simulink model "CRH2forBenchmark"  (R2014a)
settings: Solver=ode3  StartTime=0.0  StopTime=1  FixedStep=1e-5  RelTol=1e-3
PostLoadFcn:
  | , if any(exist('dsrtsu_mdlpostloadfcn', 'file') == [2, 3, 6]), try dsrtsu_mdlpostloadfcn('Execute', bdroot); catch fprintf('Error in PostLoadFcn (dsrtsu_mdlpostloadfcn) for model "%s":\n %s\n', bdroot, lasterr); end, end,
values from neighbouring files (symbols this model uses):
  Cd = 0.016    [CRH2forBenchmark.mat]
  Lm = 0.032848    [CRH2forBenchmark.mat]
  Ln = 0.002    [CRH2forBenchmark.mat]
  Lr = 0.034142    [CRH2forBenchmark.mat]
  Ls = 0.0342654    [CRH2forBenchmark.mat]
  np = 2    [CRH2forBenchmark.mat]
  Rd = 6000    [CRH2forBenchmark.mat]
  Rn = 0.2    [CRH2forBenchmark.mat]
  Rr = 0.146    [CRH2forBenchmark.mat]
  Rs = 0.144    [CRH2forBenchmark.mat]
  ts = 1e-05    [CRH2forBenchmark.mat]
undefined symbols (not defined in the file): J, KIM, KIT, KPM, KPT, phir, Ts, Vge
libraries: simulink x10
(part 2 of 3)

== system CRH2forBenchmark/InverterN/InverterTuN ==
  Tu1 : Inport
  Tu2 : Inport  Port=2
  Tu3 : Inport  Port=3
  Tu4 : Inport  Port=4
  Ia : Inport  Port=5
  U1 : Inport  Port=6
  U2 : Inport  Port=7
  InverterTuN_sfcn : S-Function  FunctionName=InverterTuN_sf  SFunctionModules=""  EnableBusSupport=off  mask{rtw_sf_name=InverterTuN_sf, showVar=off}
      mask prompts: rtw_sf_name "Simulink:masks:GenSFuncName_MP"; showVar "Simulink:masks:GenSFuncShowModuleList_MP"
      mask help: Simulink:masks:GenSFuncDesc_MD
      mask init: same as CRH2forBenchmark/DCU1/DCU1_sfcn
      settings: CopyFcn=|
      | if ~strcmp(get_param(gcb,'Linkstatus'),'none') && ...
      | ~strcmp(get_param(gcb,'Linkstatus'),'implicit')
      |   set_param(gcb,'LinkStatus','none');
      | end
      mask Help: eval('feval(''rtwprivate'',''rtwhelpview'',''rtw_sfcn_block'')');
      mask Display:
      | port_label('input',1,'Tu1');
      | port_label('input',2,'Tu2');
      | port_label('input',3,'Tu3');
      | port_label('input',4,'Tu4');
      | port_label('input',5,'Ia');
      | port_label('input',6,'U1');
      | port_label('input',7,'U2');
      | port_label('output',1,'Iu');
      | port_label('output',2,'Iz');
      | port_label('output',3,'Id');
      | port_label('output',4,'Vu');
  __InputSSForSFun__ : Subsystem
  __OutputSSForSFun__ : Subsystem
  Iu : Outport
  Iz : Outport  Port=2
  Id : Outport  Port=3
  Vu : Outport  Port=4
  wires:
  Tu1/1 -> __InputSSForSFun__/1(Tu1)
  Tu2/1 -> __InputSSForSFun__/2(Tu2)
  Tu3/1 -> __InputSSForSFun__/3(Tu3)
  Tu4/1 -> __InputSSForSFun__/4(Tu4)
  Ia/1 -> __InputSSForSFun__/5(Ia)
  U1/1 -> __InputSSForSFun__/6(U1)
  U2/1 -> __InputSSForSFun__/7(U2)
  __InputSSForSFun__/1(__UniqueOutportName__1__) -> InverterTuN_sfcn/1
  __InputSSForSFun__/2(__UniqueOutportName__2__) -> InverterTuN_sfcn/2
  __InputSSForSFun__/3(__UniqueOutportName__3__) -> InverterTuN_sfcn/3
  __InputSSForSFun__/4(__UniqueOutportName__4__) -> InverterTuN_sfcn/4
  __InputSSForSFun__/5(__UniqueOutportName__5__) -> InverterTuN_sfcn/5
  __InputSSForSFun__/6(__UniqueOutportName__6__) -> InverterTuN_sfcn/6
  __InputSSForSFun__/7(__UniqueOutportName__7__) -> InverterTuN_sfcn/7
  InverterTuN_sfcn/1 -> __OutputSSForSFun__/1(__UniqueInportName__1__)
  InverterTuN_sfcn/2 -> __OutputSSForSFun__/2(__UniqueInportName__2__)
  InverterTuN_sfcn/3 -> __OutputSSForSFun__/3(__UniqueInportName__3__)
  InverterTuN_sfcn/4 -> __OutputSSForSFun__/4(__UniqueInportName__4__)
  __OutputSSForSFun__/1(Iu) -> Iu/1
  __OutputSSForSFun__/2(Iz) -> Iz/1
  __OutputSSForSFun__/3(Id) -> Id/1
  __OutputSSForSFun__/4(Vu) -> Vu/1

== system CRH2forBenchmark/InverterN/InverterTvN ==
  Tv1 : Inport
  Tv2 : Inport  Port=2
  Tv3 : Inport  Port=3
  Tv4 : Inport  Port=4
  Ib : Inport  Port=5
  U1 : Inport  Port=6
  U2 : Inport  Port=7
  InverterTvN_sfcn : S-Function  FunctionName=InverterTvN_sf  SFunctionModules=""  EnableBusSupport=off  mask{rtw_sf_name=InverterTvN_sf, showVar=off}
      mask prompts: rtw_sf_name "Simulink:masks:GenSFuncName_MP"; showVar "Simulink:masks:GenSFuncShowModuleList_MP"
      mask help: Simulink:masks:GenSFuncDesc_MD
      mask init: same as CRH2forBenchmark/DCU1/DCU1_sfcn
      settings: CopyFcn=|
      | if ~strcmp(get_param(gcb,'Linkstatus'),'none') && ...
      | ~strcmp(get_param(gcb,'Linkstatus'),'implicit')
      |   set_param(gcb,'LinkStatus','none');
      | end
      mask Help: eval('feval(''rtwprivate'',''rtwhelpview'',''rtw_sfcn_block'')');
      mask Display:
      | port_label('input',1,'Tv1');
      | port_label('input',2,'Tv2');
      | port_label('input',3,'Tv3');
      | port_label('input',4,'Tv4');
      | port_label('input',5,'Ib');
      | port_label('input',6,'U1');
      | port_label('input',7,'U2');
      | port_label('output',1,'Iu');
      | port_label('output',2,'Iz');
      | port_label('output',3,'Id');
      | port_label('output',4,'Vv');
  __InputSSForSFun__ : Subsystem
  __OutputSSForSFun__ : Subsystem
  Iu : Outport
  Iz : Outport  Port=2
  Id : Outport  Port=3
  Vv : Outport  Port=4
  wires:
  Tv1/1 -> __InputSSForSFun__/1(Tv1)
  Tv2/1 -> __InputSSForSFun__/2(Tv2)
  Tv3/1 -> __InputSSForSFun__/3(Tv3)
  Tv4/1 -> __InputSSForSFun__/4(Tv4)
  Ib/1 -> __InputSSForSFun__/5(Ib)
  U1/1 -> __InputSSForSFun__/6(U1)
  U2/1 -> __InputSSForSFun__/7(U2)
  __InputSSForSFun__/1(__UniqueOutportName__1__) -> InverterTvN_sfcn/1
  __InputSSForSFun__/2(__UniqueOutportName__2__) -> InverterTvN_sfcn/2
  __InputSSForSFun__/3(__UniqueOutportName__3__) -> InverterTvN_sfcn/3
  __InputSSForSFun__/4(__UniqueOutportName__4__) -> InverterTvN_sfcn/4
  __InputSSForSFun__/5(__UniqueOutportName__5__) -> InverterTvN_sfcn/5
  __InputSSForSFun__/6(__UniqueOutportName__6__) -> InverterTvN_sfcn/6
  __InputSSForSFun__/7(__UniqueOutportName__7__) -> InverterTvN_sfcn/7
  InverterTvN_sfcn/1 -> __OutputSSForSFun__/1(__UniqueInportName__1__)
  InverterTvN_sfcn/2 -> __OutputSSForSFun__/2(__UniqueInportName__2__)
  InverterTvN_sfcn/3 -> __OutputSSForSFun__/3(__UniqueInportName__3__)
  InverterTvN_sfcn/4 -> __OutputSSForSFun__/4(__UniqueInportName__4__)
  __OutputSSForSFun__/1(Iu) -> Iu/1
  __OutputSSForSFun__/2(Iz) -> Iz/1
  __OutputSSForSFun__/3(Id) -> Id/1
  __OutputSSForSFun__/4(Vv) -> Vv/1

== system CRH2forBenchmark/InverterN/InverterTwN ==
  Tw1 : Inport
  Tw2 : Inport  Port=2
  Tw3 : Inport  Port=3
  Tw4 : Inport  Port=4
  Ic : Inport  Port=5
  U1 : Inport  Port=6
  U2 : Inport  Port=7
  InverterTwN_sfcn : S-Function  FunctionName=InverterTwN_sf  SFunctionModules=""  EnableBusSupport=off  mask{rtw_sf_name=InverterTwN_sf, showVar=off}
      mask prompts: rtw_sf_name "Simulink:masks:GenSFuncName_MP"; showVar "Simulink:masks:GenSFuncShowModuleList_MP"
      mask help: Simulink:masks:GenSFuncDesc_MD
      mask init: same as CRH2forBenchmark/DCU1/DCU1_sfcn
      settings: CopyFcn=|
      | if ~strcmp(get_param(gcb,'Linkstatus'),'none') && ...
      | ~strcmp(get_param(gcb,'Linkstatus'),'implicit')
      |   set_param(gcb,'LinkStatus','none');
      | end
      mask Help: eval('feval(''rtwprivate'',''rtwhelpview'',''rtw_sfcn_block'')');
      mask Display:
      | port_label('input',1,'Tw1');
      | port_label('input',2,'Tw2');
      | port_label('input',3,'Tw3');
      | port_label('input',4,'Tw4');
      | port_label('input',5,'Ic');
      | port_label('input',6,'U1');
      | port_label('input',7,'U2');
      | port_label('output',1,'Iu');
      | port_label('output',2,'Iz');
      | port_label('output',3,'Id');
      | port_label('output',4,'Vw');
  __InputSSForSFun__ : Subsystem
  __OutputSSForSFun__ : Subsystem
  Iu : Outport
  Iz : Outport  Port=2
  Id : Outport  Port=3
  Vw : Outport  Port=4
  wires:
  Tw1/1 -> __InputSSForSFun__/1(Tw1)
  Tw2/1 -> __InputSSForSFun__/2(Tw2)
  Tw3/1 -> __InputSSForSFun__/3(Tw3)
  Tw4/1 -> __InputSSForSFun__/4(Tw4)
  Ic/1 -> __InputSSForSFun__/5(Ic)
  U1/1 -> __InputSSForSFun__/6(U1)
  U2/1 -> __InputSSForSFun__/7(U2)
  __InputSSForSFun__/1(__UniqueOutportName__1__) -> InverterTwN_sfcn/1
  __InputSSForSFun__/2(__UniqueOutportName__2__) -> InverterTwN_sfcn/2
  __InputSSForSFun__/3(__UniqueOutportName__3__) -> InverterTwN_sfcn/3
  __InputSSForSFun__/4(__UniqueOutportName__4__) -> InverterTwN_sfcn/4
  __InputSSForSFun__/5(__UniqueOutportName__5__) -> InverterTwN_sfcn/5
  __InputSSForSFun__/6(__UniqueOutportName__6__) -> InverterTwN_sfcn/6
  __InputSSForSFun__/7(__UniqueOutportName__7__) -> InverterTwN_sfcn/7
  InverterTwN_sfcn/1 -> __OutputSSForSFun__/1(__UniqueInportName__1__)
  InverterTwN_sfcn/2 -> __OutputSSForSFun__/2(__UniqueInportName__2__)
  InverterTwN_sfcn/3 -> __OutputSSForSFun__/3(__UniqueInportName__3__)
  InverterTwN_sfcn/4 -> __OutputSSForSFun__/4(__UniqueInportName__4__)
  __OutputSSForSFun__/1(Iu) -> Iu/1
  __OutputSSForSFun__/2(Iz) -> Iz/1
  __OutputSSForSFun__/3(Id) -> Id/1
  __OutputSSForSFun__/4(Vw) -> Vw/1

== system CRH2forBenchmark/InverterN/Pulse ==
  note: PhaseA:1 to 4
      |
      | PhaseB:5 to 8
      |
      | PhaseC:9 to 12
  State : Inport
  Add : Sum
  Constant : Constant  Value=2
  Demux : Demux  Outputs=3
  Multiport Switch : MultiPortSwitch
  Multiport Switch1 : MultiPortSwitch
  Multiport Switch2 : MultiPortSwitch
  Mux : Mux  Inputs=3
  S =  Ud : Constant  Value=[1 1 0 0]
  S = - Ud : Constant  Value=[0 0 1 1]
  S = 0 : Constant  Value=[0 1 1 0]
  SVPWM : Outport
  wires:
  S = - Ud/1 -> Multiport Switch2/2, Multiport Switch/2, Multiport Switch1/2
  Multiport Switch/1 -> Mux/1
  S =  Ud/1 -> Multiport Switch2/4, Multiport Switch1/4, Multiport Switch/4
  Multiport Switch2/1 -> Mux/3
  Demux/1 -> Multiport Switch/1
  Mux/1 -> SVPWM/1
  Constant/1 -> Add/2
  State/1 -> Add/1
  Demux/3 -> Multiport Switch2/1
  Demux/2 -> Multiport Switch1/1
  S = 0/1 -> Multiport Switch2/3, Multiport Switch1/3, Multiport Switch/3
  Multiport Switch1/1 -> Mux/2
  Add/1 -> Demux/1

== system CRH2forBenchmark/Machine model/Normal ModelF ==
  Ua : Inport
  Ub : Inport  Port=2
  Uc : Inport  Port=3
  TL : Inport  Port=4
  MeasurementF : Subsystem  mask{sfcnParam1=J, sfcnParam2=Lm, sfcnParam3=np}
      mask prompts: sfcnParam1 "J:"; sfcnParam2 "Lm:"; sfcnParam3 "np:"
      mask help: Simulink:masks:GenSFuncDesc_MD
      mask Help: eval('feval(''rtwprivate'',''rtwhelpview'',''rtw_sfcn_block'')');
  MotorSubsystem1F : Subsystem
  MotorSubsystem2F : Subsystem
  MotorSubsystem3F : Subsystem
  MotorSubsystemF : Subsystem
  r2sF : Subsystem
      mask help: Simulink:masks:GenSFuncDesc_MD
      mask Help: eval('feval(''rtwprivate'',''rtwhelpview'',''rtw_sfcn_block'')');
  Te0 : Outport
  Isabc0 : Outport  Port=2
  w : Outport  Port=3
  wires:
  MeasurementF/3(Isabc) -> Isabc0/1
  MotorSubsystem2F/2(ψrα) -> MotorSubsystem3F/2(ψrα), MotorSubsystemF/1(ψrα)
  MotorSubsystem1F/2(ψsβ) -> MotorSubsystem3F/1(ψsβ)
  MotorSubsystem2F/1(irα) -> MeasurementF/3(irα)
  MeasurementF/1(Te) -> Te0/1
  TL/1 -> MeasurementF/5(TL)
  MotorSubsystemF/2(ψsα) -> MotorSubsystem2F/1(ψsα)
  r2sF/1(Usα) -> MotorSubsystemF/2(Usα)
  MotorSubsystem3F/2(ψrβ) -> MotorSubsystem1F/1(ψrβ), MotorSubsystem2F/2(ψrβ)
  MotorSubsystemF/1(isα) -> MeasurementF/1(isα)
  r2sF/2(Usβ) -> MotorSubsystem1F/2(Usβ)
  MotorSubsystem3F/1(irβ) -> MeasurementF/4(irβ)
  MeasurementF/2(ω) -> MotorSubsystem2F/3(ω), MotorSubsystem3F/3(ω), w/1
  MotorSubsystem1F/1(isβ) -> MeasurementF/2(isβ)
  Uc/1 -> r2sF/3(Uc)
  Ub/1 -> r2sF/2(Ub)
  Ua/1 -> r2sF/1(Ua)

== system CRH2forBenchmark/Machine model1/Normal ModelN ==
  Ua : Inport
  Ub : Inport  Port=2
  Uc : Inport  Port=3
  TL : Inport  Port=4
  MeasurementN : Subsystem  mask{sfcnParam1=J, sfcnParam2=Lm, sfcnParam3=np}
      mask prompts: sfcnParam1 "J:"; sfcnParam2 "Lm:"; sfcnParam3 "np:"
      mask help: Simulink:masks:GenSFuncDesc_MD
      mask Help: eval('feval(''rtwprivate'',''rtwhelpview'',''rtw_sfcn_block'')');
  MotorSubsystem1N : Subsystem
  MotorSubsystem2N : Subsystem
  MotorSubsystem3N : Subsystem
  MotorSubsystemN : Subsystem
  r2sN : Subsystem
      mask help: Simulink:masks:GenSFuncDesc_MD
      mask Help: eval('feval(''rtwprivate'',''rtwhelpview'',''rtw_sfcn_block'')');
  Te0 : Outport
  Isabc0 : Outport  Port=2
  w : Outport  Port=3
  wires:
  MeasurementN/3(Isabc) -> Isabc0/1
  MotorSubsystem2N/2(ψrα) -> MotorSubsystem3N/2(ψrα), MotorSubsystemN/1(ψrα)
  MotorSubsystem1N/2(ψsβ) -> MotorSubsystem3N/1(ψsβ)
  MotorSubsystem2N/1(irα) -> MeasurementN/3(irα)
  MeasurementN/1(Te) -> Te0/1
  TL/1 -> MeasurementN/5(TL)
  MotorSubsystemN/2(ψsα) -> MotorSubsystem2N/1(ψsα)
  r2sN/1(Usα) -> MotorSubsystemN/2(Usα)
  MotorSubsystem3N/2(ψrβ) -> MotorSubsystem1N/1(ψrβ), MotorSubsystem2N/2(ψrβ)
  MotorSubsystemN/1(isα) -> MeasurementN/1(isα)
  r2sN/2(Usβ) -> MotorSubsystem1N/2(Usβ)
  MotorSubsystem3N/1(irβ) -> MeasurementN/4(irβ)
  MeasurementN/2(ω) -> MotorSubsystem2N/3(ω), MotorSubsystem3N/3(ω), w/1
  MotorSubsystem1N/1(isβ) -> MeasurementN/2(isβ)
  Uc/1 -> r2sN/3(Uc)
  Ub/1 -> r2sN/2(Ub)
  Ua/1 -> r2sN/1(Ua)

== system CRH2forBenchmark/TFI1/TFI1Sub ==
  Nomal : Inport
  Outside Signal : Inport  Port=2
  Add : Sum
  Band-Limited White Noise : simulink/Sources/Band-Limited White Noise  Cov=NoiseFault(1)  Ts=NoiseFault(2)  seed=NoiseFault(3)
  Logic Operation : Subsystem
  Noise0 : Constant  Value=0
  NoiseAdd : Sum  Inputs=++|
  NoiseSelec : Constant  Value=NoiseSelec
  Product : Product
  Switch : Switch  Criteria=u2 ~= 0
  TFI : Subsystem
  Out : Outport
  wires:
  NoiseSelec/1 -> Switch/2
  [Selector] -> Logic Operation/1(Selector)
  TFI/2(Selector) -> [Selector]
  Product/1 -> Logic Operation/3(Mux)
  TFI/1(Fault Singal) -> [Fault]
  Noise0/1 -> Switch/3
  Add/1 -> Logic Operation/2(Add)
  Nomal/1 -> Logic Operation/4(Normal), Product/1, Add/1
  Logic Operation/1(Out) -> NoiseAdd/2
  NoiseAdd/1 -> Out/1
  [Fault] -> Product/2, Add/2, Logic Operation/5(Fault)
  Band-Limited White Noise/1 -> Switch/1
  Switch/1 -> NoiseAdd/1
  Outside Signal/1 -> TFI/1(Outside Signal)

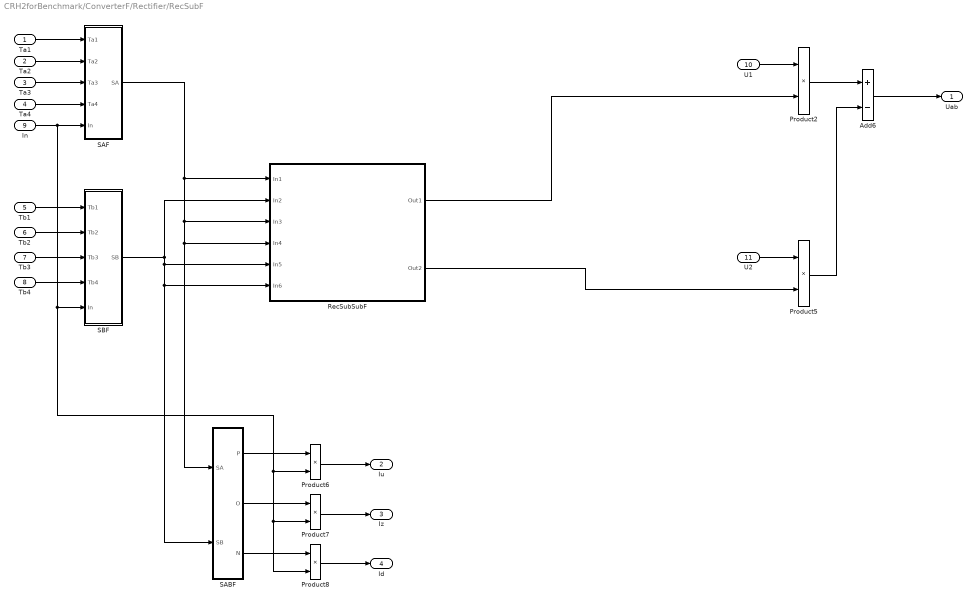
== system CRH2forBenchmark/ConverterF/Rectifier/RecSubF ==
  Ta1 : Inport
  Ta2 : Inport  Port=2
  Ta3 : Inport  Port=3
  Ta4 : Inport  Port=4
  Tb1 : Inport  Port=5
  Tb2 : Inport  Port=6
  Tb3 : Inport  Port=7
  Tb4 : Inport  Port=8
  In : Inport  Port=9
  U1 : Inport  Port=10
  U2 : Inport  Port=11
  Add6 : Sum  Inputs=+-  SampleTime=ts
  Product{2,5..8} (5 alike) : Product  SampleTime=ts
  RecSubSubF : Subsystem
      mask help: Simulink:masks:GenSFuncDesc_MD
      mask Help: eval('feval(''rtwprivate'',''rtwhelpview'',''rtw_sfcn_block'')');
  SABF : Subsystem
      mask help: Simulink:masks:GenSFuncDesc_MD
      mask Help: eval('feval(''rtwprivate'',''rtwhelpview'',''rtw_sfcn_block'')');
  SAF : Subsystem
      mask help: Simulink:masks:GenSFuncDesc_MD
      mask Help: eval('feval(''rtwprivate'',''rtwhelpview'',''rtw_sfcn_block'')');
  SBF : Subsystem
      mask help: Simulink:masks:GenSFuncDesc_MD
      mask Help: eval('feval(''rtwprivate'',''rtwhelpview'',''rtw_sfcn_block'')');
  Uab : Outport
  Iu : Outport  Port=2
  Iz : Outport  Port=3
  Id : Outport  Port=4
  wires:
  In/1 -> SAF/5(In), SBF/5(In), Product7/2, Product8/2, Product6/2
  Tb3/1 -> SBF/3(Tb3)
  U2/1 -> Product5/1
  Product2/1 -> Add6/1
  SAF/1(SA) -> RecSubSubF/1(In1), RecSubSubF/3(In3), RecSubSubF/4(In4), SABF/1(SA)
  U1/1 -> Product2/1
  Ta3/1 -> SAF/3(Ta3)
  Product5/1 -> Add6/2
  Tb1/1 -> SBF/1(Tb1)
  Add6/1 -> Uab/1
  Ta2/1 -> SAF/2(Ta2)
  Tb2/1 -> SBF/2(Tb2)
  SBF/1(SB) -> RecSubSubF/2(In2), RecSubSubF/5(In5), RecSubSubF/6(In6), SABF/2(SB)
  Tb4/1 -> SBF/4(Tb4)
  Ta1/1 -> SAF/1(Ta1)
  Ta4/1 -> SAF/4(Ta4)
  SABF/3(N) -> Product8/1
  SABF/2(O) -> Product7/1
  SABF/1(P) -> Product6/1
  Product6/1 -> Iu/1
  Product7/1 -> Iz/1
  Product8/1 -> Id/1
  RecSubSubF/1(Out1) -> Product2/2
  RecSubSubF/2(Out2) -> Product5/2

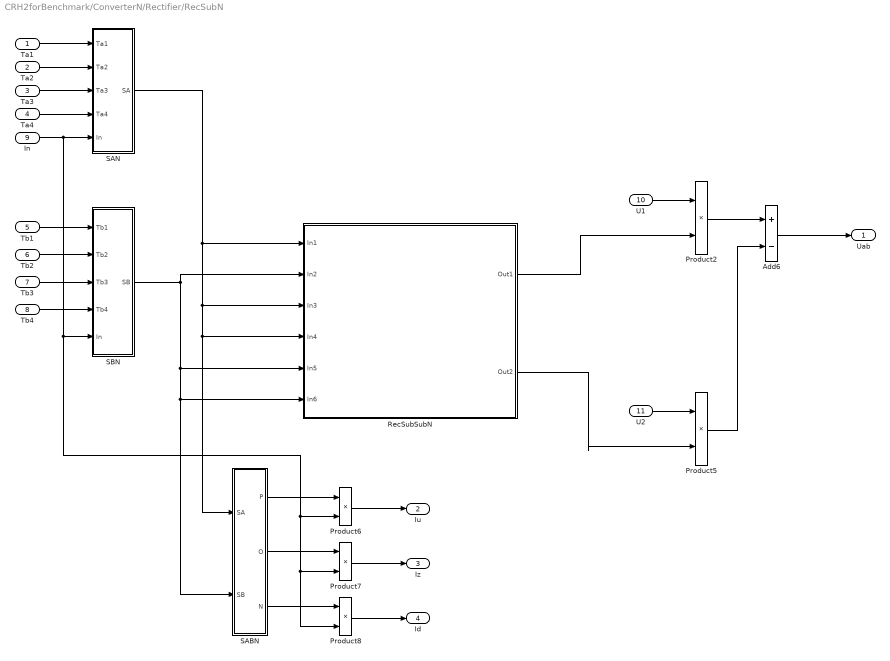
== system CRH2forBenchmark/ConverterN/Rectifier/RecSubN ==
  Ta1 : Inport
  Ta2 : Inport  Port=2
  Ta3 : Inport  Port=3
  Ta4 : Inport  Port=4
  Tb1 : Inport  Port=5
  Tb2 : Inport  Port=6
  Tb3 : Inport  Port=7
  Tb4 : Inport  Port=8
  In : Inport  Port=9
  U1 : Inport  Port=10
  U2 : Inport  Port=11
  Add6 : Sum  Inputs=+-  SampleTime=ts
  Product{2,5..8} (5 alike) : Product  SampleTime=ts
  RecSubSubN : Subsystem
      mask help: Simulink:masks:GenSFuncDesc_MD
      mask Help: eval('feval(''rtwprivate'',''rtwhelpview'',''rtw_sfcn_block'')');
  SABN : Subsystem
      mask help: Simulink:masks:GenSFuncDesc_MD
      mask Help: eval('feval(''rtwprivate'',''rtwhelpview'',''rtw_sfcn_block'')');
  SAN : Subsystem
      mask help: Simulink:masks:GenSFuncDesc_MD
      mask Help: eval('feval(''rtwprivate'',''rtwhelpview'',''rtw_sfcn_block'')');
  SBN : Subsystem
      mask help: Simulink:masks:GenSFuncDesc_MD
      mask Help: eval('feval(''rtwprivate'',''rtwhelpview'',''rtw_sfcn_block'')');
  Uab : Outport
  Iu : Outport  Port=2
  Iz : Outport  Port=3
  Id : Outport  Port=4
  wires:
  Product8/1 -> Id/1
  Product7/1 -> Iz/1
  Product6/1 -> Iu/1
  SABN/1(P) -> Product6/1
  SABN/2(O) -> Product7/1
  SABN/3(N) -> Product8/1
  Ta4/1 -> SAN/4(Ta4)
  Ta1/1 -> SAN/1(Ta1)
  Tb4/1 -> SBN/4(Tb4)
  SBN/1(SB) -> RecSubSubN/2(In2), RecSubSubN/5(In5), RecSubSubN/6(In6), SABN/2(SB)
  Tb2/1 -> SBN/2(Tb2)
  Ta2/1 -> SAN/2(Ta2)
  Add6/1 -> Uab/1
  Tb1/1 -> SBN/1(Tb1)
  Product5/1 -> Add6/2
  Ta3/1 -> SAN/3(Ta3)
  U1/1 -> Product2/1
  SAN/1(SA) -> RecSubSubN/1(In1), RecSubSubN/3(In3), RecSubSubN/4(In4), SABN/1(SA)
  Product2/1 -> Add6/1
  U2/1 -> Product5/1
  Tb3/1 -> SBN/3(Tb3)
  In/1 -> SAN/5(In), SBN/5(In), Product6/2, Product8/2, Product7/2
  RecSubSubN/1(Out1) -> Product2/2
  RecSubSubN/2(Out2) -> Product5/2

== system CRH2forBenchmark/InverterF/InverterTuF/__InputSSForSFun__ ==
  Tu1 : Inport
  Tu2 : Inport  Port=2
  Tu3 : Inport  Port=3
  Tu4 : Inport  Port=4
  Ia : Inport  Port=5
  U1 : Inport  Port=6
  U2 : Inport  Port=7
  __UniqueOutportName__1__ : Outport
  __UniqueOutportName__2__ : Outport  Port=2
  __UniqueOutportName__3__ : Outport  Port=3
  __UniqueOutportName__4__ : Outport  Port=4
  __UniqueOutportName__5__ : Outport  Port=5
  __UniqueOutportName__6__ : Outport  Port=6
  __UniqueOutportName__7__ : Outport  Port=7
  wires:
  Tu1/1 -> __UniqueOutportName__1__/1
  Tu2/1 -> __UniqueOutportName__2__/1
  Tu3/1 -> __UniqueOutportName__3__/1
  Tu4/1 -> __UniqueOutportName__4__/1
  Ia/1 -> __UniqueOutportName__5__/1
  U1/1 -> __UniqueOutportName__6__/1
  U2/1 -> __UniqueOutportName__7__/1

== system CRH2forBenchmark/InverterF/InverterTuF/__OutputSSForSFun__ ==
  __UniqueInportName__1__ : Inport
  __UniqueInportName__2__ : Inport  Port=2
  __UniqueInportName__3__ : Inport  Port=3
  __UniqueInportName__4__ : Inport  Port=4
  Iu : Outport
  Iz : Outport  Port=2
  Id : Outport  Port=3
  Vu : Outport  Port=4
  wires:
  __UniqueInportName__1__/1 -> Iu/1
  __UniqueInportName__2__/1 -> Iz/1
  __UniqueInportName__3__/1 -> Id/1
  __UniqueInportName__4__/1 -> Vu/1

== system CRH2forBenchmark/InverterF/InverterTvF/__InputSSForSFun__ ==
  Tv1 : Inport
  Tv2 : Inport  Port=2
  Tv3 : Inport  Port=3
  Tv4 : Inport  Port=4
  Ib : Inport  Port=5
  U1 : Inport  Port=6
  U2 : Inport  Port=7
  __UniqueOutportName__1__ : Outport
  __UniqueOutportName__2__ : Outport  Port=2
  __UniqueOutportName__3__ : Outport  Port=3
  __UniqueOutportName__4__ : Outport  Port=4
  __UniqueOutportName__5__ : Outport  Port=5
  __UniqueOutportName__6__ : Outport  Port=6
  __UniqueOutportName__7__ : Outport  Port=7
  wires:
  Tv1/1 -> __UniqueOutportName__1__/1
  Tv2/1 -> __UniqueOutportName__2__/1
  Tv3/1 -> __UniqueOutportName__3__/1
  Tv4/1 -> __UniqueOutportName__4__/1
  Ib/1 -> __UniqueOutportName__5__/1
  U1/1 -> __UniqueOutportName__6__/1
  U2/1 -> __UniqueOutportName__7__/1

== system CRH2forBenchmark/InverterF/InverterTvF/__OutputSSForSFun__ ==
  __UniqueInportName__1__ : Inport
  __UniqueInportName__2__ : Inport  Port=2
  __UniqueInportName__3__ : Inport  Port=3
  __UniqueInportName__4__ : Inport  Port=4
  Iu : Outport
  Iz : Outport  Port=2
  Id : Outport  Port=3
  Vv : Outport  Port=4
  wires:
  __UniqueInportName__1__/1 -> Iu/1
  __UniqueInportName__2__/1 -> Iz/1
  __UniqueInportName__3__/1 -> Id/1
  __UniqueInportName__4__/1 -> Vv/1

== system CRH2forBenchmark/InverterF/InverterTwF/__InputSSForSFun__ ==
  Tw1 : Inport
  Tw2 : Inport  Port=2
  Tw3 : Inport  Port=3
  Tw4 : Inport  Port=4
  Ic : Inport  Port=5
  U1 : Inport  Port=6
  U2 : Inport  Port=7
  __UniqueOutportName__1__ : Outport
  __UniqueOutportName__2__ : Outport  Port=2
  __UniqueOutportName__3__ : Outport  Port=3
  __UniqueOutportName__4__ : Outport  Port=4
  __UniqueOutportName__5__ : Outport  Port=5
  __UniqueOutportName__6__ : Outport  Port=6
  __UniqueOutportName__7__ : Outport  Port=7
  wires:
  Tw1/1 -> __UniqueOutportName__1__/1
  Tw2/1 -> __UniqueOutportName__2__/1
  Tw3/1 -> __UniqueOutportName__3__/1
  Tw4/1 -> __UniqueOutportName__4__/1
  Ic/1 -> __UniqueOutportName__5__/1
  U1/1 -> __UniqueOutportName__6__/1
  U2/1 -> __UniqueOutportName__7__/1

== system CRH2forBenchmark/InverterF/InverterTwF/__OutputSSForSFun__ ==
  __UniqueInportName__1__ : Inport
  __UniqueInportName__2__ : Inport  Port=2
  __UniqueInportName__3__ : Inport  Port=3
  __UniqueInportName__4__ : Inport  Port=4
  Iu : Outport
  Iz : Outport  Port=2
  Id : Outport  Port=3
  Vw : Outport  Port=4
  wires:
  __UniqueInportName__1__/1 -> Iu/1
  __UniqueInportName__2__/1 -> Iz/1
  __UniqueInportName__3__/1 -> Id/1
  __UniqueInportName__4__/1 -> Vw/1

== system CRH2forBenchmark/InverterN/InverterTuN/__InputSSForSFun__ ==
  Tu1 : Inport
  Tu2 : Inport  Port=2
  Tu3 : Inport  Port=3
  Tu4 : Inport  Port=4
  Ia : Inport  Port=5
  U1 : Inport  Port=6
  U2 : Inport  Port=7
  __UniqueOutportName__1__ : Outport
  __UniqueOutportName__2__ : Outport  Port=2
  __UniqueOutportName__3__ : Outport  Port=3
  __UniqueOutportName__4__ : Outport  Port=4
  __UniqueOutportName__5__ : Outport  Port=5
  __UniqueOutportName__6__ : Outport  Port=6
  __UniqueOutportName__7__ : Outport  Port=7
  wires:
  Tu1/1 -> __UniqueOutportName__1__/1
  Tu2/1 -> __UniqueOutportName__2__/1
  Tu3/1 -> __UniqueOutportName__3__/1
  Tu4/1 -> __UniqueOutportName__4__/1
  Ia/1 -> __UniqueOutportName__5__/1
  U1/1 -> __UniqueOutportName__6__/1
  U2/1 -> __UniqueOutportName__7__/1

== system CRH2forBenchmark/InverterN/InverterTuN/__OutputSSForSFun__ ==
  __UniqueInportName__1__ : Inport
  __UniqueInportName__2__ : Inport  Port=2
  __UniqueInportName__3__ : Inport  Port=3
  __UniqueInportName__4__ : Inport  Port=4
  Iu : Outport
  Iz : Outport  Port=2
  Id : Outport  Port=3
  Vu : Outport  Port=4
  wires:
  __UniqueInportName__1__/1 -> Iu/1
  __UniqueInportName__2__/1 -> Iz/1
  __UniqueInportName__3__/1 -> Id/1
  __UniqueInportName__4__/1 -> Vu/1

== system CRH2forBenchmark/InverterN/InverterTvN/__InputSSForSFun__ ==
  Tv1 : Inport
  Tv2 : Inport  Port=2
  Tv3 : Inport  Port=3
  Tv4 : Inport  Port=4
  Ib : Inport  Port=5
  U1 : Inport  Port=6
  U2 : Inport  Port=7
  __UniqueOutportName__1__ : Outport
  __UniqueOutportName__2__ : Outport  Port=2
  __UniqueOutportName__3__ : Outport  Port=3
  __UniqueOutportName__4__ : Outport  Port=4
  __UniqueOutportName__5__ : Outport  Port=5
  __UniqueOutportName__6__ : Outport  Port=6
  __UniqueOutportName__7__ : Outport  Port=7
  wires:
  Tv1/1 -> __UniqueOutportName__1__/1
  Tv2/1 -> __UniqueOutportName__2__/1
  Tv3/1 -> __UniqueOutportName__3__/1
  Tv4/1 -> __UniqueOutportName__4__/1
  Ib/1 -> __UniqueOutportName__5__/1
  U1/1 -> __UniqueOutportName__6__/1
  U2/1 -> __UniqueOutportName__7__/1

== system CRH2forBenchmark/InverterN/InverterTvN/__OutputSSForSFun__ ==
  __UniqueInportName__1__ : Inport
  __UniqueInportName__2__ : Inport  Port=2
  __UniqueInportName__3__ : Inport  Port=3
  __UniqueInportName__4__ : Inport  Port=4
  Iu : Outport
  Iz : Outport  Port=2
  Id : Outport  Port=3
  Vv : Outport  Port=4
  wires:
  __UniqueInportName__1__/1 -> Iu/1
  __UniqueInportName__2__/1 -> Iz/1
  __UniqueInportName__3__/1 -> Id/1
  __UniqueInportName__4__/1 -> Vv/1

== system CRH2forBenchmark/InverterN/InverterTwN/__InputSSForSFun__ ==
  Tw1 : Inport
  Tw2 : Inport  Port=2
  Tw3 : Inport  Port=3
  Tw4 : Inport  Port=4
  Ic : Inport  Port=5
  U1 : Inport  Port=6
  U2 : Inport  Port=7
  __UniqueOutportName__1__ : Outport
  __UniqueOutportName__2__ : Outport  Port=2
  __UniqueOutportName__3__ : Outport  Port=3
  __UniqueOutportName__4__ : Outport  Port=4
  __UniqueOutportName__5__ : Outport  Port=5
  __UniqueOutportName__6__ : Outport  Port=6
  __UniqueOutportName__7__ : Outport  Port=7
  wires:
  Tw1/1 -> __UniqueOutportName__1__/1
  Tw2/1 -> __UniqueOutportName__2__/1
  Tw3/1 -> __UniqueOutportName__3__/1
  Tw4/1 -> __UniqueOutportName__4__/1
  Ic/1 -> __UniqueOutportName__5__/1
  U1/1 -> __UniqueOutportName__6__/1
  U2/1 -> __UniqueOutportName__7__/1

== system CRH2forBenchmark/InverterN/InverterTwN/__OutputSSForSFun__ ==
  __UniqueInportName__1__ : Inport
  __UniqueInportName__2__ : Inport  Port=2
  __UniqueInportName__3__ : Inport  Port=3
  __UniqueInportName__4__ : Inport  Port=4
  Iu : Outport
  Iz : Outport  Port=2
  Id : Outport  Port=3
  Vw : Outport  Port=4
  wires:
  __UniqueInportName__1__/1 -> Iu/1
  __UniqueInportName__2__/1 -> Iz/1
  __UniqueInportName__3__/1 -> Id/1
  __UniqueInportName__4__/1 -> Vw/1

== system CRH2forBenchmark/Machine model/Normal ModelF/MeasurementF ==
  isα : Inport
  isβ : Inport  Port=2
  irα : Inport  Port=3
  irβ : Inport  Port=4
  TL : Inport  Port=5
  MeasurementF_sfcn : S-Function  FunctionName=MeasurementF_sf  Parameters=sfcnParam1, sfcnParam2, sfcnParam3  SFunctionModules=""  EnableBusSupport=off  mask{rtw_sf_name=MeasurementF_sf, showVar=off, sfcnParam1=sfcnParam1, sfcnParam2=sfcnParam2, sfcnParam3=sfcnParam3}
      mask prompts: rtw_sf_name "Simulink:masks:GenSFuncName_MP"; showVar "Simulink:masks:GenSFuncShowModuleList_MP"; sfcnParam1 "J:"; sfcnParam2 "Lm:"; sfcnParam3 "np:"
      mask help: Simulink:masks:GenSFuncDesc_MD
      mask init: same as CRH2forBenchmark/DCU1/DCU1_sfcn
      settings: CopyFcn=|
      | if ~strcmp(get_param(gcb,'Linkstatus'),'none') && ...
      | ~strcmp(get_param(gcb,'Linkstatus'),'implicit')
      |   set_param(gcb,'LinkStatus','none');
      | end
      mask Help: eval('feval(''rtwprivate'',''rtwhelpview'',''rtw_sfcn_block'')');
      mask Display:
      | port_label('input',1,'isα');
      | port_label('input',2,'isβ');
      | port_label('input',3,'irα');
      | port_label('input',4,'irβ');
      | port_label('input',5,'TL');
      | port_label('output',1,'Te');
      | port_label('output',2,'ω');
      | port_label('output',3,'Isabc');
  __InputSSForSFun__ : Subsystem
  __OutputSSForSFun__ : Subsystem
  Te : Outport
  ω : Outport  Port=2
  Isabc : Outport  Port=3
  wires:
  isα/1 -> __InputSSForSFun__/1(isα)
  isβ/1 -> __InputSSForSFun__/2(isβ)
  irα/1 -> __InputSSForSFun__/3(irα)
  irβ/1 -> __InputSSForSFun__/4(irβ)
  TL/1 -> __InputSSForSFun__/5(TL)
  __InputSSForSFun__/1(__UniqueOutportName__1__) -> MeasurementF_sfcn/1
  __InputSSForSFun__/2(__UniqueOutportName__2__) -> MeasurementF_sfcn/2
  __InputSSForSFun__/3(__UniqueOutportName__3__) -> MeasurementF_sfcn/3
  __InputSSForSFun__/4(__UniqueOutportName__4__) -> MeasurementF_sfcn/4
  __InputSSForSFun__/5(__UniqueOutportName__5__) -> MeasurementF_sfcn/5
  MeasurementF_sfcn/1 -> __OutputSSForSFun__/1(__UniqueInportName__1__)
  MeasurementF_sfcn/2 -> __OutputSSForSFun__/2(__UniqueInportName__2__)
  MeasurementF_sfcn/3 -> __OutputSSForSFun__/3(__UniqueInportName__3__)
  __OutputSSForSFun__/1(Te) -> Te/1
  __OutputSSForSFun__/2(ω) -> ω/1
  __OutputSSForSFun__/3(Isabc) -> Isabc/1

== system CRH2forBenchmark/Machine model/Normal ModelF/MotorSubsystem1F ==
  ψrβ : Inport
  Usβ : Inport  Port=2
  MotorSubsystem1FSub : Subsystem
  isβ : Outport
  ψsβ : Outport  Port=2
  wires:
  ψrβ/1 -> MotorSubsystem1FSub/1(ψrβ)
  Usβ/1 -> MotorSubsystem1FSub/2(Usβ)
  MotorSubsystem1FSub/1(isβ) -> isβ/1
  MotorSubsystem1FSub/2(ψsβ) -> ψsβ/1

== system CRH2forBenchmark/Machine model/Normal ModelF/MotorSubsystem2F ==
  ψsα : Inport
  ψrβ : Inport  Port=2
  ω : Inport  Port=3
  MotorSubsystem2FSub : Subsystem
  irα : Outport
  ψrα : Outport  Port=2
  wires:
  ψsα/1 -> MotorSubsystem2FSub/1(ψsα)
  ψrβ/1 -> MotorSubsystem2FSub/2(ψrβ)
  ω/1 -> MotorSubsystem2FSub/3(ω)
  MotorSubsystem2FSub/1(irα) -> irα/1
  MotorSubsystem2FSub/2(ψrα) -> ψrα/1

== system CRH2forBenchmark/Machine model/Normal ModelF/MotorSubsystem3F ==
  ψsβ : Inport
  ψrα : Inport  Port=2
  ω : Inport  Port=3
  MotorSubsystem3FSub : Subsystem
  irβ : Outport
  ψrβ : Outport  Port=2
  wires:
  ψsβ/1 -> MotorSubsystem3FSub/1(ψsβ)
  ψrα/1 -> MotorSubsystem3FSub/2(ψrα)
  ω/1 -> MotorSubsystem3FSub/3(ω)
  MotorSubsystem3FSub/1(irβ) -> irβ/1
  MotorSubsystem3FSub/2(ψrβ) -> ψrβ/1

== system CRH2forBenchmark/Machine model/Normal ModelF/MotorSubsystemF ==
  ψrα : Inport
  Usα : Inport  Port=2
  MotorSubsystemFSub : Subsystem
  isα : Outport
  ψsα : Outport  Port=2
  wires:
  ψrα/1 -> MotorSubsystemFSub/1(ψrα)
  Usα/1 -> MotorSubsystemFSub/2(Usα)
  MotorSubsystemFSub/1(isα) -> isα/1
  MotorSubsystemFSub/2(ψsα) -> ψsα/1

== system CRH2forBenchmark/Machine model/Normal ModelF/r2sF ==
  Ua : Inport
  Ub : Inport  Port=2
  Uc : Inport  Port=3
  __InputSSForSFun__ : Subsystem
  __OutputSSForSFun__ : Subsystem
  r2sF_sfcn : S-Function  FunctionName=r2sF_sf  SFunctionModules=""  EnableBusSupport=off  mask{rtw_sf_name=r2sF_sf, showVar=off}
      mask prompts: rtw_sf_name "Simulink:masks:GenSFuncName_MP"; showVar "Simulink:masks:GenSFuncShowModuleList_MP"
      mask help: Simulink:masks:GenSFuncDesc_MD
      mask init: same as CRH2forBenchmark/DCU1/DCU1_sfcn
      settings: CopyFcn=|
      | if ~strcmp(get_param(gcb,'Linkstatus'),'none') && ...
      | ~strcmp(get_param(gcb,'Linkstatus'),'implicit')
      |   set_param(gcb,'LinkStatus','none');
      | end
      mask Help: eval('feval(''rtwprivate'',''rtwhelpview'',''rtw_sfcn_block'')');
      mask Display:
      | port_label('input',1,'Ua');
      | port_label('input',2,'Ub');
      | port_label('input',3,'Uc');
      | port_label('output',1,'Usα');
      | port_label('output',2,'Usβ');
  Usα : Outport
  Usβ : Outport  Port=2
  wires:
  Ua/1 -> __InputSSForSFun__/1(Ua)
  Ub/1 -> __InputSSForSFun__/2(Ub)
  Uc/1 -> __InputSSForSFun__/3(Uc)
  __InputSSForSFun__/1(__UniqueOutportName__1__) -> r2sF_sfcn/1
  __InputSSForSFun__/2(__UniqueOutportName__2__) -> r2sF_sfcn/2
  __InputSSForSFun__/3(__UniqueOutportName__3__) -> r2sF_sfcn/3
  r2sF_sfcn/1 -> __OutputSSForSFun__/1(__UniqueInportName__1__)
  r2sF_sfcn/2 -> __OutputSSForSFun__/2(__UniqueInportName__2__)
  __OutputSSForSFun__/1(Usα) -> Usα/1
  __OutputSSForSFun__/2(Usβ) -> Usβ/1

== system CRH2forBenchmark/Machine model1/Normal ModelN/MeasurementN ==
  isα : Inport
  isβ : Inport  Port=2
  irα : Inport  Port=3
  irβ : Inport  Port=4
  TL : Inport  Port=5
  MeasurementN_sfcn : S-Function  FunctionName=MeasurementN_sf  Parameters=sfcnParam1, sfcnParam2, sfcnParam3  SFunctionModules=""  EnableBusSupport=off  mask{rtw_sf_name=MeasurementN_sf, showVar=off, sfcnParam1=sfcnParam1, sfcnParam2=sfcnParam2, sfcnParam3=sfcnParam3}
      mask prompts: rtw_sf_name "Simulink:masks:GenSFuncName_MP"; showVar "Simulink:masks:GenSFuncShowModuleList_MP"; sfcnParam1 "J:"; sfcnParam2 "Lm:"; sfcnParam3 "np:"
      mask help: Simulink:masks:GenSFuncDesc_MD
      mask init: same as CRH2forBenchmark/DCU1/DCU1_sfcn
      settings: CopyFcn=|
      | if ~strcmp(get_param(gcb,'Linkstatus'),'none') && ...
      | ~strcmp(get_param(gcb,'Linkstatus'),'implicit')
      |   set_param(gcb,'LinkStatus','none');
      | end
      mask Help: eval('feval(''rtwprivate'',''rtwhelpview'',''rtw_sfcn_block'')');
      mask Display:
      | port_label('input',1,'isα');
      | port_label('input',2,'isβ');
      | port_label('input',3,'irα');
      | port_label('input',4,'irβ');
      | port_label('input',5,'TL');
      | port_label('output',1,'Te');
      | port_label('output',2,'ω');
      | port_label('output',3,'Isabc');
  __InputSSForSFun__ : Subsystem
  __OutputSSForSFun__ : Subsystem
  Te : Outport
  ω : Outport  Port=2
  Isabc : Outport  Port=3
  wires:
  isα/1 -> __InputSSForSFun__/1(isα)
  isβ/1 -> __InputSSForSFun__/2(isβ)
  irα/1 -> __InputSSForSFun__/3(irα)
  irβ/1 -> __InputSSForSFun__/4(irβ)
  TL/1 -> __InputSSForSFun__/5(TL)
  __InputSSForSFun__/1(__UniqueOutportName__1__) -> MeasurementN_sfcn/1
  __InputSSForSFun__/2(__UniqueOutportName__2__) -> MeasurementN_sfcn/2
  __InputSSForSFun__/3(__UniqueOutportName__3__) -> MeasurementN_sfcn/3
  __InputSSForSFun__/4(__UniqueOutportName__4__) -> MeasurementN_sfcn/4
  __InputSSForSFun__/5(__UniqueOutportName__5__) -> MeasurementN_sfcn/5
  MeasurementN_sfcn/1 -> __OutputSSForSFun__/1(__UniqueInportName__1__)
  MeasurementN_sfcn/2 -> __OutputSSForSFun__/2(__UniqueInportName__2__)
  MeasurementN_sfcn/3 -> __OutputSSForSFun__/3(__UniqueInportName__3__)
  __OutputSSForSFun__/1(Te) -> Te/1
  __OutputSSForSFun__/2(ω) -> ω/1
  __OutputSSForSFun__/3(Isabc) -> Isabc/1

== system CRH2forBenchmark/Machine model1/Normal ModelN/MotorSubsystem1N ==
  ψrβ : Inport
  Usβ : Inport  Port=2
  MotorSubsystem1NSub : Subsystem
  isβ : Outport
  ψsβ : Outport  Port=2
  wires:
  ψrβ/1 -> MotorSubsystem1NSub/1(ψrβ)
  Usβ/1 -> MotorSubsystem1NSub/2(Usβ)
  MotorSubsystem1NSub/1(isβ) -> isβ/1
  MotorSubsystem1NSub/2(ψsβ) -> ψsβ/1

== system CRH2forBenchmark/Machine model1/Normal ModelN/MotorSubsystem2N ==
  ψsα : Inport
  ψrβ : Inport  Port=2
  ω : Inport  Port=3
  MotorSubsystem2NSub : Subsystem
  irα : Outport
  ψrα : Outport  Port=2
  wires:
  ψsα/1 -> MotorSubsystem2NSub/1(ψsα)
  ψrβ/1 -> MotorSubsystem2NSub/2(ψrβ)
  ω/1 -> MotorSubsystem2NSub/3(ω)
  MotorSubsystem2NSub/1(irα) -> irα/1
  MotorSubsystem2NSub/2(ψrα) -> ψrα/1

== system CRH2forBenchmark/Machine model1/Normal ModelN/MotorSubsystem3N ==
  ψsβ : Inport
  ψrα : Inport  Port=2
  ω : Inport  Port=3
  MotorSubsystem3NSub : Subsystem
  irβ : Outport
  ψrβ : Outport  Port=2
  wires:
  ψsβ/1 -> MotorSubsystem3NSub/1(ψsβ)
  ψrα/1 -> MotorSubsystem3NSub/2(ψrα)
  ω/1 -> MotorSubsystem3NSub/3(ω)
  MotorSubsystem3NSub/1(irβ) -> irβ/1
  MotorSubsystem3NSub/2(ψrβ) -> ψrβ/1

== system CRH2forBenchmark/Machine model1/Normal ModelN/MotorSubsystemN ==
  ψrα : Inport
  Usα : Inport  Port=2
  MotorSubsystemNSub : Subsystem
  isα : Outport
  ψsα : Outport  Port=2
  wires:
  ψrα/1 -> MotorSubsystemNSub/1(ψrα)
  Usα/1 -> MotorSubsystemNSub/2(Usα)
  MotorSubsystemNSub/1(isα) -> isα/1
  MotorSubsystemNSub/2(ψsα) -> ψsα/1

== system CRH2forBenchmark/Machine model1/Normal ModelN/r2sN ==
  Ua : Inport
  Ub : Inport  Port=2
  Uc : Inport  Port=3
  __InputSSForSFun__ : Subsystem
  __OutputSSForSFun__ : Subsystem
  r2sN_sfcn : S-Function  FunctionName=r2sN_sf  SFunctionModules=""  EnableBusSupport=off  mask{rtw_sf_name=r2sN_sf, showVar=off}
      mask prompts: rtw_sf_name "Simulink:masks:GenSFuncName_MP"; showVar "Simulink:masks:GenSFuncShowModuleList_MP"
      mask help: Simulink:masks:GenSFuncDesc_MD
      mask init: same as CRH2forBenchmark/DCU1/DCU1_sfcn
      settings: CopyFcn=|
      | if ~strcmp(get_param(gcb,'Linkstatus'),'none') && ...
      | ~strcmp(get_param(gcb,'Linkstatus'),'implicit')
      |   set_param(gcb,'LinkStatus','none');
      | end
      mask Help: eval('feval(''rtwprivate'',''rtwhelpview'',''rtw_sfcn_block'')');
      mask Display:
      | port_label('input',1,'Ua');
      | port_label('input',2,'Ub');
      | port_label('input',3,'Uc');
      | port_label('output',1,'Usα');
      | port_label('output',2,'Usβ');
  Usα : Outport
  Usβ : Outport  Port=2
  wires:
  Ua/1 -> __InputSSForSFun__/1(Ua)
  Ub/1 -> __InputSSForSFun__/2(Ub)
  Uc/1 -> __InputSSForSFun__/3(Uc)
  __InputSSForSFun__/1(__UniqueOutportName__1__) -> r2sN_sfcn/1
  __InputSSForSFun__/2(__UniqueOutportName__2__) -> r2sN_sfcn/2
  __InputSSForSFun__/3(__UniqueOutportName__3__) -> r2sN_sfcn/3
  r2sN_sfcn/1 -> __OutputSSForSFun__/1(__UniqueInportName__1__)
  r2sN_sfcn/2 -> __OutputSSForSFun__/2(__UniqueInportName__2__)
  __OutputSSForSFun__/1(Usα) -> Usα/1
  __OutputSSForSFun__/2(Usβ) -> Usβ/1

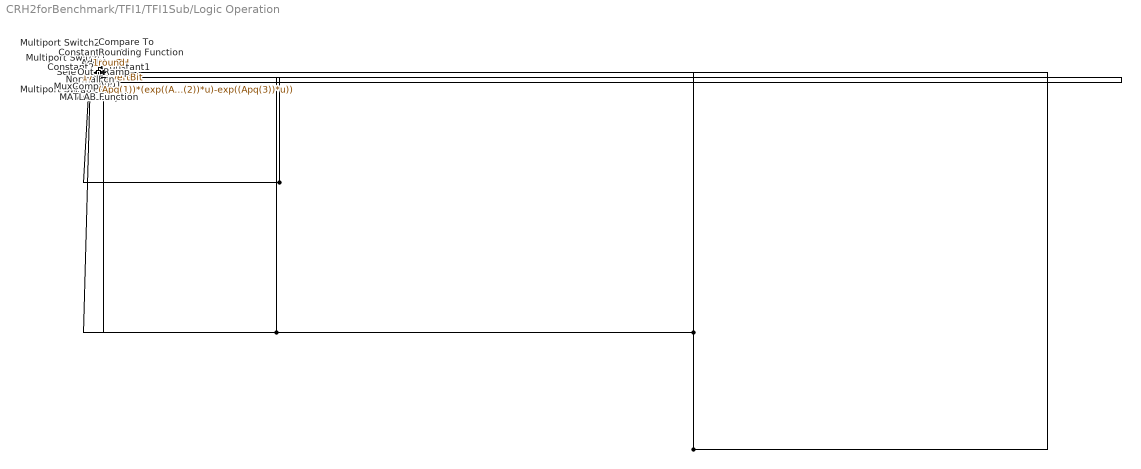
== system CRH2forBenchmark/TFI1/TFI1Sub/Logic Operation ==
  Selector : Inport
  Add : Inport  Port=2
  Mux : Inport  Port=3
  Normal : Inport  Port=4
  Fault : Inport  Port=5
  Add1 : Sum  Inputs=+-
  AddComp : Subsystem
  Compare To Constant : simulink/Logic and Bit Operations/Compare To Constant  relop=>=  const=TH  OutDataTypeStr=boolean
  Constant : Constant
  Constant1 : Constant  Value=InvertBit
  Constant2 : Constant  Value=17
  FaultSelec : Step  Time=FaultInjectionTime  Before=1  After=FaultType  SampleTime=0
  Fcn : Fcn  Expr=(Apq(1))*(exp((Apq(2))*u)-exp((Apq(3))*u))
  MATLAB Function : MATLAB Function  TreatAsAtomicUnit=on  SystemSampleTime=Register_Ts
  Multiport Switch : MultiPortSwitch  DataPortOrder=Zero-based contiguous  Inputs=2
  Multiport Switch1 : MultiPortSwitch  DataPortOrder=Specify indices  Inputs=2  DataPortIndices={[1,2,5],3,4}
  Multiport Switch2 : MultiPortSwitch  Inputs=8
  MuxComp : Subsystem
  Ramp : simulink/Sources/Ramp  slope=1  start=FaultInjectionTime  X0=0
  Rounding Function : Rounding  Operator=round  SampleTime=Register_Ts
  Out : Outport
  wires:
  Fault/1 -> Multiport Switch2/9
  Constant2/1 -> Add1/1
  Add1/1 -> MATLAB Function/2(Num)
  MATLAB Function/1(y) -> Multiport Switch1/4
  Constant1/1 -> Add1/2
  Rounding Function/1 -> MATLAB Function/1(x)
  MuxComp/2(Out2) -> Multiport Switch2/7
  MuxComp/1(Out1) -> Multiport Switch2/6
  AddComp/2(Out2) -> Multiport Switch2/4
  AddComp/1(Out1) -> Multiport Switch2/3
  Normal/1 -> Multiport Switch2/8
  Multiport Switch/1 -> Multiport Switch1/3
  Compare To Constant/1 -> Multiport Switch/1
  Fcn/1 -> Compare To Constant/1
  Ramp/1 -> Fcn/1
  Constant/1 -> Multiport Switch/3
  Multiport Switch2/1 -> Multiport Switch1/2, Multiport Switch/2, Rounding Function/1
  FaultSelec/1 -> Multiport Switch1/1
  Multiport Switch1/1 -> Out/1
  Add/1 -> Multiport Switch2/2, AddComp/1(Add)
  Selector/1 -> Multiport Switch2/1
  Mux/1 -> Multiport Switch2/5, MuxComp/1(Mux)

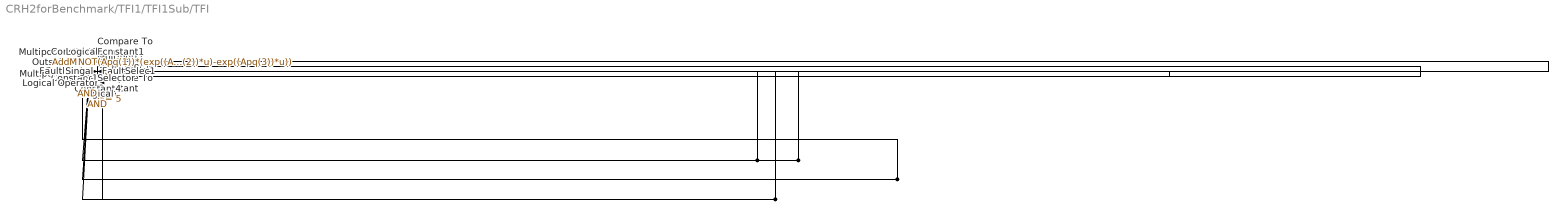
== system CRH2forBenchmark/TFI1/TFI1Sub/TFI ==
  Outside Signal : Inport
  " " : Constant  Value=7
  "  " : Constant
  "   " : Constant  Value=4
  "   1" : Constant  Value=8
  0 : Constant  Value=0
  Compare To Constant : simulink/Logic and Bit Operations/Compare To Constant  relop===  const=5  OutDataTypeStr=boolean
  Compare To Constant1 : simulink/Logic and Bit Operations/Compare To Constant  relop===  const=5  OutDataTypeStr=boolean
  Constant1 : Constant  Value=5
  Constant2 : Constant  Value=AddMux-1
  Constant3 : Constant  Value=2
  Constant4 : Constant  Value=6
  FaultSelec : Step  Time=FaultInjectionTime  Before=1  After=FaultType  SampleTime=0
  FaultSelec1 : Step  Time=FaultInjectionTime  Before=1  After=FaultType  SampleTime=0
  Fcn : Fcn  Expr=(Apq(1))*(exp((Apq(2))*u)-exp((Apq(3))*u))
  Logical : Logic  Operator=NOT  AllPortsSameDT=off  OutDataTypeStr=boolean
  "Logical " : Logic  AllPortsSameDT=off  OutDataTypeStr=boolean
  Logical Operator : Logic  AllPortsSameDT=off  OutDataTypeStr=boolean
  Multiport : MultiPortSwitch  DataPortOrder=Zero-based contiguous  Inputs=2
  Multiport Switch : MultiPortSwitch  DataPortOrder=Specify indices  Inputs=4  DataPortIndices={[1,3,4],2,5}
  Multiport Switch1 : MultiPortSwitch  DataPortOrder=Specify indices  Inputs=4  DataPortIndices={[1,3,4],2,5,6}
  "Multiport  " : MultiPortSwitch  DataPortOrder=Zero-based contiguous  Inputs=2
  Multiport1 : MultiPortSwitch  DataPortOrder=Zero-based contiguous  Inputs=2
  Ramp : simulink/Sources/Ramp  slope=1  start=FaultInjectionTime  X0=0
  Fault Singal : Outport
  Selector : Outport  Port=2
  wires:
  "   1"/1 -> Multiport Switch1/5
  Constant1/1 -> Multiport1/2
  Constant4/1 -> Multiport1/3
  Compare To Constant1/1 -> Multiport1/1
  Outside Signal/1 -> Multiport Switch/4
  "   "/1 -> Multiport Switch1/4
  Logical/1 -> "Logical "/1
  "Logical "/1 -> "Multiport  "/1
  Multiport/1 -> "Multiport  "/2
  Constant3/1 -> "Multiport  "/3
  "Multiport  "/1 -> Multiport Switch1/1
  Multiport1/1 -> Multiport/3
  Logical Operator/1 -> Multiport/1
  Compare To Constant/1 -> Logical Operator/2, "Logical "/2
  Constant2/1 -> Logical Operator/1, Logical/1, Compare To Constant1/1
  FaultSelec1/1 -> Multiport/2, Compare To Constant/1
  "  "/1 -> Multiport Switch1/3
  " "/1 -> Multiport Switch1/2
  Fcn/1 -> Multiport Switch/3
  0/1 -> Multiport Switch/2
  Multiport Switch1/1 -> Selector/1
  FaultSelec/1 -> Multiport Switch/1
  Multiport Switch/1 -> Fault Singal/1
  Ramp/1 -> Fcn/1

== system CRH2forBenchmark/ConverterF/Rectifier/RecSubF/RecSubSubF ==
  In1 : Inport
  In2 : Inport  Port=2
  In3 : Inport  Port=3
  In4 : Inport  Port=4
  In5 : Inport  Port=5
  In6 : Inport  Port=6
  RecSubSubF_sfcn : S-Function  FunctionName=RecSubSubF_sf  SFunctionModules=""  EnableBusSupport=off  mask{rtw_sf_name=RecSubSubF_sf, showVar=off}
      mask prompts: rtw_sf_name "Simulink:masks:GenSFuncName_MP"; showVar "Simulink:masks:GenSFuncShowModuleList_MP"
      mask help: Simulink:masks:GenSFuncDesc_MD
      mask init: same as CRH2forBenchmark/DCU1/DCU1_sfcn
      settings: CopyFcn=|
      | if ~strcmp(get_param(gcb,'Linkstatus'),'none') && ...
      | ~strcmp(get_param(gcb,'Linkstatus'),'implicit')
      |   set_param(gcb,'LinkStatus','none');
      | end
      mask Help: eval('feval(''rtwprivate'',''rtwhelpview'',''rtw_sfcn_block'')');
      mask Display:
      | port_label('input',1,'In1');
      | port_label('input',2,'In2');
      | port_label('input',3,'In3');
      | port_label('input',4,'In4');
      | port_label('input',5,'In5');
      | port_label('input',6,'In6');
      | port_label('output',1,'Out1');
      | port_label('output',2,'Out2');
  __InputSSForSFun__ : Subsystem
  __OutputSSForSFun__ : Subsystem
  Out1 : Outport
  Out2 : Outport  Port=2
  wires:
  In1/1 -> __InputSSForSFun__/1(In1)
  In2/1 -> __InputSSForSFun__/2(In2)
  In3/1 -> __InputSSForSFun__/3(In3)
  In4/1 -> __InputSSForSFun__/4(In4)
  In5/1 -> __InputSSForSFun__/5(In5)
  In6/1 -> __InputSSForSFun__/6(In6)
  __InputSSForSFun__/1(__UniqueOutportName__1__) -> RecSubSubF_sfcn/1
  __InputSSForSFun__/2(__UniqueOutportName__2__) -> RecSubSubF_sfcn/2
  __InputSSForSFun__/3(__UniqueOutportName__3__) -> RecSubSubF_sfcn/3
  __InputSSForSFun__/4(__UniqueOutportName__4__) -> RecSubSubF_sfcn/4
  __InputSSForSFun__/5(__UniqueOutportName__5__) -> RecSubSubF_sfcn/5
  __InputSSForSFun__/6(__UniqueOutportName__6__) -> RecSubSubF_sfcn/6
  RecSubSubF_sfcn/1 -> __OutputSSForSFun__/1(__UniqueInportName__1__)
  RecSubSubF_sfcn/2 -> __OutputSSForSFun__/2(__UniqueInportName__2__)
  __OutputSSForSFun__/1(Out1) -> Out1/1
  __OutputSSForSFun__/2(Out2) -> Out2/1

== system CRH2forBenchmark/ConverterF/Rectifier/RecSubF/SABF ==
  SA : Inport
  SB : Inport  Port=2
  SABF_sfcn : S-Function  FunctionName=SABF_sf  SFunctionModules=""  EnableBusSupport=off  mask{rtw_sf_name=SABF_sf, showVar=off}
      mask prompts: rtw_sf_name "Simulink:masks:GenSFuncName_MP"; showVar "Simulink:masks:GenSFuncShowModuleList_MP"
      mask help: Simulink:masks:GenSFuncDesc_MD
      mask init: same as CRH2forBenchmark/DCU1/DCU1_sfcn
      settings: CopyFcn=|
      | if ~strcmp(get_param(gcb,'Linkstatus'),'none') && ...
      | ~strcmp(get_param(gcb,'Linkstatus'),'implicit')
      |   set_param(gcb,'LinkStatus','none');
      | end
      mask Help: eval('feval(''rtwprivate'',''rtwhelpview'',''rtw_sfcn_block'')');
      mask Display:
      | port_label('input',1,'SA');
      | port_label('input',2,'SB');
      | port_label('output',1,'P');
      | port_label('output',2,'O');
      | port_label('output',3,'N');
  __InputSSForSFun__ : Subsystem
  __OutputSSForSFun__ : Subsystem
  P : Outport
  O : Outport  Port=2
  N : Outport  Port=3
  wires:
  SA/1 -> __InputSSForSFun__/1(SA)
  SB/1 -> __InputSSForSFun__/2(SB)
  __InputSSForSFun__/1(__UniqueOutportName__1__) -> SABF_sfcn/1
  __InputSSForSFun__/2(__UniqueOutportName__2__) -> SABF_sfcn/2
  SABF_sfcn/1 -> __OutputSSForSFun__/1(__UniqueInportName__1__)
  SABF_sfcn/2 -> __OutputSSForSFun__/2(__UniqueInportName__2__)
  SABF_sfcn/3 -> __OutputSSForSFun__/3(__UniqueInportName__3__)
  __OutputSSForSFun__/1(P) -> P/1
  __OutputSSForSFun__/2(O) -> O/1
  __OutputSSForSFun__/3(N) -> N/1

== system CRH2forBenchmark/ConverterF/Rectifier/RecSubF/SAF ==
  Ta1 : Inport
  Ta2 : Inport  Port=2
  Ta3 : Inport  Port=3
  Ta4 : Inport  Port=4
  In : Inport  Port=5
  SAF_sfcn : S-Function  FunctionName=SAF_sf  SFunctionModules=""  EnableBusSupport=off  mask{rtw_sf_name=SAF_sf, showVar=off}
      mask prompts: rtw_sf_name "Simulink:masks:GenSFuncName_MP"; showVar "Simulink:masks:GenSFuncShowModuleList_MP"
      mask help: Simulink:masks:GenSFuncDesc_MD
      mask init: same as CRH2forBenchmark/DCU1/DCU1_sfcn
      settings: CopyFcn=|
      | if ~strcmp(get_param(gcb,'Linkstatus'),'none') && ...
      | ~strcmp(get_param(gcb,'Linkstatus'),'implicit')
      |   set_param(gcb,'LinkStatus','none');
      | end
      mask Help: eval('feval(''rtwprivate'',''rtwhelpview'',''rtw_sfcn_block'')');
      mask Display:
      | port_label('input',1,'Ta1');
      | port_label('input',2,'Ta2');
      | port_label('input',3,'Ta3');
      | port_label('input',4,'Ta4');
      | port_label('input',5,'In');
      | port_label('output',1,'SA');
  __InputSSForSFun__ : Subsystem
  __OutputSSForSFun__ : Subsystem
  SA : Outport
  wires:
  Ta1/1 -> __InputSSForSFun__/1(Ta1)
  Ta2/1 -> __InputSSForSFun__/2(Ta2)
  Ta3/1 -> __InputSSForSFun__/3(Ta3)
  Ta4/1 -> __InputSSForSFun__/4(Ta4)
  In/1 -> __InputSSForSFun__/5(In)
  __InputSSForSFun__/1(__UniqueOutportName__1__) -> SAF_sfcn/1
  __InputSSForSFun__/2(__UniqueOutportName__2__) -> SAF_sfcn/2
  __InputSSForSFun__/3(__UniqueOutportName__3__) -> SAF_sfcn/3
  __InputSSForSFun__/4(__UniqueOutportName__4__) -> SAF_sfcn/4
  __InputSSForSFun__/5(__UniqueOutportName__5__) -> SAF_sfcn/5
  SAF_sfcn/1 -> __OutputSSForSFun__/1(__UniqueInportName__1__)
  __OutputSSForSFun__/1(SA) -> SA/1

== system CRH2forBenchmark/ConverterF/Rectifier/RecSubF/SBF ==
  Tb1 : Inport
  Tb2 : Inport  Port=2
  Tb3 : Inport  Port=3
  Tb4 : Inport  Port=4
  In : Inport  Port=5
  SBF_sfcn : S-Function  FunctionName=SBF_sf  SFunctionModules=""  EnableBusSupport=off  mask{rtw_sf_name=SBF_sf, showVar=off}
      mask prompts: rtw_sf_name "Simulink:masks:GenSFuncName_MP"; showVar "Simulink:masks:GenSFuncShowModuleList_MP"
      mask help: Simulink:masks:GenSFuncDesc_MD
      mask init: same as CRH2forBenchmark/DCU1/DCU1_sfcn
      settings: CopyFcn=|
      | if ~strcmp(get_param(gcb,'Linkstatus'),'none') && ...
      | ~strcmp(get_param(gcb,'Linkstatus'),'implicit')
      |   set_param(gcb,'LinkStatus','none');
      | end
      mask Help: eval('feval(''rtwprivate'',''rtwhelpview'',''rtw_sfcn_block'')');
      mask Display:
      | port_label('input',1,'Tb1');
      | port_label('input',2,'Tb2');
      | port_label('input',3,'Tb3');
      | port_label('input',4,'Tb4');
      | port_label('input',5,'In');
      | port_label('output',1,'SB');
  __InputSSForSFun__ : Subsystem
  __OutputSSForSFun__ : Subsystem
  SB : Outport
  wires:
  Tb1/1 -> __InputSSForSFun__/1(Tb1)
  Tb2/1 -> __InputSSForSFun__/2(Tb2)
  Tb3/1 -> __InputSSForSFun__/3(Tb3)
  Tb4/1 -> __InputSSForSFun__/4(Tb4)
  In/1 -> __InputSSForSFun__/5(In)
  __InputSSForSFun__/1(__UniqueOutportName__1__) -> SBF_sfcn/1
  __InputSSForSFun__/2(__UniqueOutportName__2__) -> SBF_sfcn/2
  __InputSSForSFun__/3(__UniqueOutportName__3__) -> SBF_sfcn/3
  __InputSSForSFun__/4(__UniqueOutportName__4__) -> SBF_sfcn/4
  __InputSSForSFun__/5(__UniqueOutportName__5__) -> SBF_sfcn/5
  SBF_sfcn/1 -> __OutputSSForSFun__/1(__UniqueInportName__1__)
  __OutputSSForSFun__/1(SB) -> SB/1

== system CRH2forBenchmark/ConverterN/Rectifier/RecSubN/RecSubSubN ==
  In1 : Inport
  In2 : Inport  Port=2
  In3 : Inport  Port=3
  In4 : Inport  Port=4
  In5 : Inport  Port=5
  In6 : Inport  Port=6
  RecSubSubN_sfcn : S-Function  FunctionName=RecSubSubN_sf  SFunctionModules=""  EnableBusSupport=off  mask{rtw_sf_name=RecSubSubN_sf, showVar=off}
      mask prompts: rtw_sf_name "Simulink:masks:GenSFuncName_MP"; showVar "Simulink:masks:GenSFuncShowModuleList_MP"
      mask help: Simulink:masks:GenSFuncDesc_MD
      mask init: same as CRH2forBenchmark/DCU1/DCU1_sfcn
      settings: CopyFcn=|
      | if ~strcmp(get_param(gcb,'Linkstatus'),'none') && ...
      | ~strcmp(get_param(gcb,'Linkstatus'),'implicit')
      |   set_param(gcb,'LinkStatus','none');
      | end
      mask Help: eval('feval(''rtwprivate'',''rtwhelpview'',''rtw_sfcn_block'')');
      mask Display:
      | port_label('input',1,'In1');
      | port_label('input',2,'In2');
      | port_label('input',3,'In3');
      | port_label('input',4,'In4');
      | port_label('input',5,'In5');
      | port_label('input',6,'In6');
      | port_label('output',1,'Out1');
      | port_label('output',2,'Out2');
  __InputSSForSFun__ : Subsystem
  __OutputSSForSFun__ : Subsystem
  Out1 : Outport
  Out2 : Outport  Port=2
  wires:
  In1/1 -> __InputSSForSFun__/1(In1)
  In2/1 -> __InputSSForSFun__/2(In2)
  In3/1 -> __InputSSForSFun__/3(In3)
  In4/1 -> __InputSSForSFun__/4(In4)
  In5/1 -> __InputSSForSFun__/5(In5)
  In6/1 -> __InputSSForSFun__/6(In6)
  __InputSSForSFun__/1(__UniqueOutportName__1__) -> RecSubSubN_sfcn/1
  __InputSSForSFun__/2(__UniqueOutportName__2__) -> RecSubSubN_sfcn/2
  __InputSSForSFun__/3(__UniqueOutportName__3__) -> RecSubSubN_sfcn/3
  __InputSSForSFun__/4(__UniqueOutportName__4__) -> RecSubSubN_sfcn/4
  __InputSSForSFun__/5(__UniqueOutportName__5__) -> RecSubSubN_sfcn/5
  __InputSSForSFun__/6(__UniqueOutportName__6__) -> RecSubSubN_sfcn/6
  RecSubSubN_sfcn/1 -> __OutputSSForSFun__/1(__UniqueInportName__1__)
  RecSubSubN_sfcn/2 -> __OutputSSForSFun__/2(__UniqueInportName__2__)
  __OutputSSForSFun__/1(Out1) -> Out1/1
  __OutputSSForSFun__/2(Out2) -> Out2/1
